simulink model "offboard_SSC_simscape"  (R2025b)
settings: Solver=ode23t  StartTime=0.0  StopTime=0.3  RelTol=1e-3
undefined symbols (not defined in the file): PLL_3ph__class, V_ref
libraries: fl_lib x39, nesl_utility x20, ee_lib x9, simulink x6, eeTransforms x2, batteryecm_lib x1, eeSinusoidalMeasurement x1
(part 1 of 2)
settings Model: SimulationMode=accelerator  Creator=a6039  LastModifiedBy=axz5845
settings SolverCC: AlgebraicLoopSolver=TrustRegion
settings DataIOCC: Decimation=50
settings DebuggingCC: SaveWithParameterizedLinksMsg=none  UnconnectedInputMsg=warning  UnconnectedOutputMsg=warning  UnconnectedLineMsg=warning
settings ModelReferenceCC: EnableRefExpFcnMdlSchedulingChecks=on
settings RTWCC: GPUComputeCapability=3.5  DLArmComputeVersion=19.05

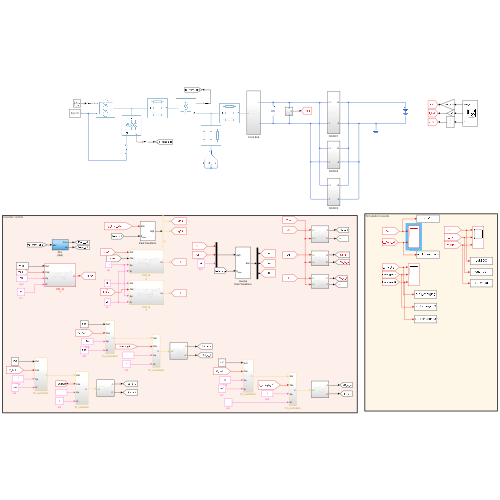
[thumbnail: Simulink's stored preview of the top-level diagram]
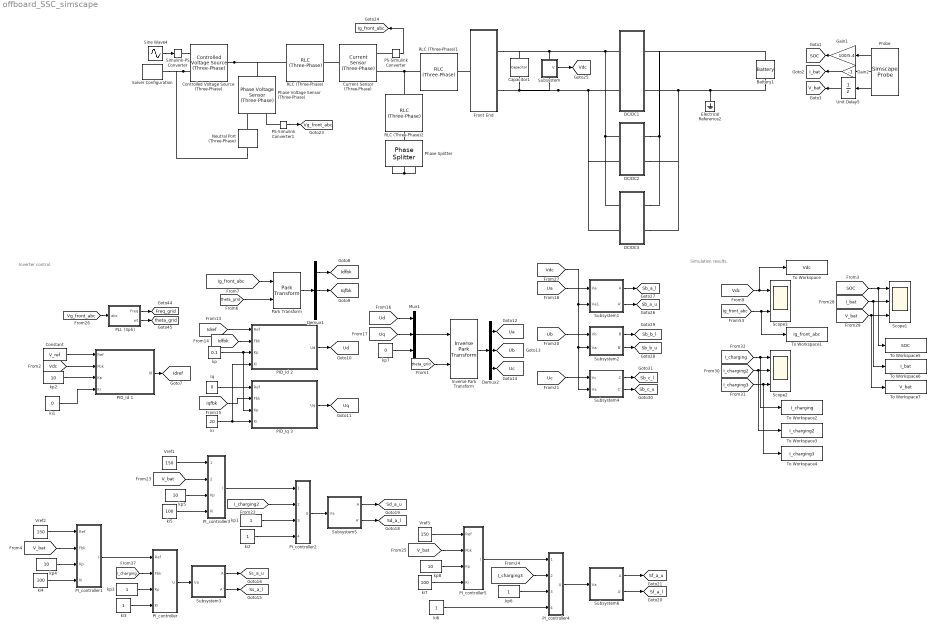
== system offboard_SSC_simscape ==
  note: Simulation results.
  note: Inverter control
  Battery1 : batteryecm_lib/Battery  Vnom=400 V  prm_dir=simscape.enum.battery.prm_dir.disabled  R1_dis=2 Ohm  R1_ch=2 Ohm  R1=2 Ohm  prm_AH=simscape.enum.battery.prm_AH.finite  AH=5.4 A*hr  V1=95 V  AH1=0.54 A*hr  prm_R2=simscape.enum.battery.prm_R2.disabled  R2=2000 Ohm  Tmeas=298.15 K  charge_measurement_port=simscape.enum.battery.enable.no  prm_dyn=simscape.enum.battery.prm_dyn.off  Rp1=0.005 Ohm  tau1=30 s  Rp2=0.005 Ohm  tau2=30 s  Rp3=0.005 Ohm  tau3=30 s  Rp4=0.005 Ohm  tau4=30 s  Rp5=0.005 Ohm  tau5=30 s  prm_fade=simscape.enum.battery.prm_fade.disabled  N_fade=100  AH_fade=45 A*hr  R1_fade=2.02 Ohm  R1_ch_fade=2.02 Ohm  V1_fade=10.35 V  prm_age=simscape.enum.battery.prm_age.disabled  prm_age_OCV=simscape.enum.battery.prm_age_OCV.OCV  OCV_age=0.9  SOC_age=60  Tmeas_age=298.15 K  delta_time_age_vec=[0] d  temperature_age_vec=[273] K  OCV_scaling_age=2.2134e6  OCV_offset_age=1.632e6  temp_exp_age=0.515833569 V  t_exp_age=0.75  Vnom_T2=12 V  R1_T2=2.2 Ohm  R1_T2_dis=2.2 Ohm  R1_T2_ch=2.2 Ohm  V1_T2=11.4 V  R2_T2=2200 Ohm  Rp1_T2=0.005 Ohm  tau1_T2=30 s  Rp2_T2=0.005 Ohm  tau2_T2=30 s  Rp3_T2=0.005 Ohm  tau3_T2=30 s  Rp4_T2=0.005 Ohm  tau4_T2=30 s  Rp5_T2=0.005 Ohm  tau5_T2=30 s  Tmeas2=273.15 K  thermal_port=simscape.enum.thermaleffects.omit  thermal_mass=30000 J/K  i_specify=off  i_priority=None  i=0 A  i_nominal_specify=off  i_nominal_value=1  i_nominal_unit=A  v_specify=off  v_priority=None  v=0 V  v_nominal_specify=off  v_nominal_value=1  v_nominal_unit=V  charge_specify=on  charge_priority=High  charge=0.54 A*hr  charge_nominal_specify=off  charge_nominal_value=1  charge_nominal_unit=A*hr  num_cycles_specify=off  num_cycles_priority=High  num_cycles=0  num_cycles_nominal_specify=off  num_cycles_nominal_value=1  num_cycles_nominal_unit=1  temperature_specify=off  temperature_priority=High  temperature=298.15 K  temperature_nominal_specify=off  temperature_nominal_value=1  temperature_nominal_unit=K
  Capacitor1 : fl_lib/Electrical/Electrical Elements/Capacitor  c=2 mF  r=1e-9 Ohm  g=0 1/Ohm  i_specify=off  i_priority=None  i=0 A  i_nominal_specify=off  i_nominal_value=1  i_nominal_unit=A  v_specify=off  v_priority=None  v=900 V  v_nominal_specify=off  v_nominal_value=1  v_nominal_unit=V  vc_specify=off  vc_priority=High  vc=900 V  vc_nominal_specify=off  vc_nominal_value=1  vc_nominal_unit=V
  Constant : Constant  Value=V_ref
  Controlled Voltage Source (Three-Phase) : ee_lib/Sources/Controlled Voltage Source (Three-Phase)  input_option=ee.enum.inputType.instantaneous  FRated=60 Hz
      settings: InternalSimscapePortConfiguration="{\"Bottom\":[],\"Left\":[{\"id\":\"S\",\"label\":\"S\",\"type\":\"input\"},{\"id\":\"n\",\"label\":\"n\",\"type\":\"foundation.electrical.electrical\"}],\"Right\":[{\"id\":\"N\",\"label\":\"~\",\"type\":\"foundation.electrical.three_phase\"}],\"Top\":[]}"
  Current Sensor (Three-Phase) : ee_lib/Sensors & Transducers/Current Sensor (Three-Phase)
  DC/DC1 : Subsystem
  DC/DC2 : Subsystem
  DC/DC3 : Subsystem
  Demux1 : Demux  Outputs=3
  Demux2 : Demux  Outputs=3
  Electrical Reference2 : fl_lib/Electrical/Electrical Elements/Electrical Reference
  Front End : Subsystem
  Gain1 : Gain  Gain=100/5.4
  Gain2 : Gain  Gain=-1
  Inverse Park Transform : eeTransforms/Inverse Park Transform  AxisAlignment=Q-axis  PowerInvariant=off
      settings: LibrarySourceBlock=|
      | ee_sl_lib/Mathematical
      | Transforms/Inverse
      | Park Transform
  Iq : Constant  Value=0
  Mux1 : Mux  Inputs=3
  Neutral Port (Three-Phase) : ee_lib/Connectors & References/Neutral Port (Three-Phase)  G_parasitic=1e-12 1/Ohm
      settings: InternalSimscapePortConfiguration="{\"Bottom\":[],\"Left\":[{\"id\":\"N\",\"label\":\"~\",\"type\":\"foundation.electrical.three_phase\"}],\"Right\":[{\"id\":\"n\",\"label\":\"n\",\"type\":\"foundation.electrical.electrical\"}],\"Top\":[]}"
  PID_Id 1 : Subsystem
  PID_Id 2 : Subsystem
  PID_Iq 3 : Subsystem
  PI_controller : Subsystem
  PI_controller1 : Subsystem
  PI_controller2 : Subsystem
  PI_controller3 : Subsystem
  PI_controller4 : Subsystem
  PI_controller5 : Subsystem
  PLL (3ph) : Subsystem
  PS-Simulink Converter : nesl_utility/PS-Simulink Converter  PhysicalDomain=network_engine_domain  SubClassName=ps_output  LeftPortType=input  RightPortType=output  PseudoPeriodic=off  Frequencies=[]  VectorFormat=inherit  Unit=inherit  AffineConversion=off
  PS-Simulink Converter1 : nesl_utility/PS-Simulink Converter  PhysicalDomain=network_engine_domain  SubClassName=ps_output  LeftPortType=input  RightPortType=output  PseudoPeriodic=off  Frequencies=[]  VectorFormat=inherit  Unit=inherit  AffineConversion=off
  Park Transform : eeTransforms/Park Transform  AxisAlignment=Q-axis  PowerInvariant=off
      settings: LibrarySourceBlock=|
      | ee_sl_lib/Mathematical
      | Transforms/Park Transform
  Phase Splitter : ee_lib/Connectors & References/Phase Splitter
  Phase Voltage Sensor (Three-Phase) : ee_lib/Sensors & Transducers/Phase Voltage Sensor (Three-Phase)
  Probe : SimscapeProbe  BoundBlock=1149  Variables="{\"charge\":{\"Probing\":\"ON\"},\"i\":{\"Probing\":\"ON\"},\"v\":{\"Probing\":\"ON\"}}"
  RLC (Three-Phase) : ee_lib/Passive/RLC Assemblies/RLC (Three-Phase)  port_option=ee.enum.threePhasePort.composite  component_structure=ee.enum.rlc.structure.SeriesRL  R=1 Ohm  L=1e-6 H  C=1e-6 F  R_parasitic=0 Ohm  G_parasitic=0 1/Ohm  IL_specify=off  IL_priority=High  IL=[0, 0, 0] A  IL_nominal_specify=off  IL_nominal_value=1  IL_nominal_unit=A  VC_specify=off  VC_priority=High  VC=[0, 0, 0] V  VC_nominal_specify=off  VC_nominal_value=1  VC_nominal_unit=V
      settings: InternalSimscapePortConfiguration="{\"Bottom\":[],\"Left\":[{\"id\":\"N1\",\"label\":\"~1\",\"type\":\"foundation.electrical.three_phase\"}],\"Right\":[{\"id\":\"N2\",\"label\":\"~2\",\"type\":\"foundation.electrical.three_phase\"}],\"Top\":[]}"
  RLC (Three-Phase)1 : ee_lib/Passive/RLC Assemblies/RLC (Three-Phase)  port_option=ee.enum.threePhasePort.composite  component_structure=ee.enum.rlc.structure.SeriesRL  R=1e-3 Ohm  L=250e-6 H  C=1e-6 F  R_parasitic=0 Ohm  G_parasitic=0 1/Ohm  IL_specify=off  IL_priority=High  IL=[0, 0, 0] A  IL_nominal_specify=off  IL_nominal_value=1  IL_nominal_unit=A  VC_specify=off  VC_priority=High  VC=[0, 0, 0] V  VC_nominal_specify=off  VC_nominal_value=1  VC_nominal_unit=V
      settings: InternalSimscapePortConfiguration="{\"Bottom\":[],\"Left\":[{\"id\":\"N1\",\"label\":\"~1\",\"type\":\"foundation.electrical.three_phase\"}],\"Right\":[{\"id\":\"N2\",\"label\":\"~2\",\"type\":\"foundation.electrical.three_phase\"}],\"Top\":[]}"
  RLC (Three-Phase)2 : ee_lib/Passive/RLC Assemblies/RLC (Three-Phase)  port_option=ee.enum.threePhasePort.composite  component_structure=ee.enum.rlc.structure.SeriesRC  R=1e-9 Ohm  L=80e-6 H  C=8.8e-6 F  R_parasitic=0 Ohm  G_parasitic=0 1/Ohm  IL_specify=off  IL_priority=High  IL=[0, 0, 0] A  IL_nominal_specify=off  IL_nominal_value=1  IL_nominal_unit=A  VC_specify=off  VC_priority=High  VC=[0, 0, 0] V  VC_nominal_specify=off  VC_nominal_value=1  VC_nominal_unit=V
      settings: InternalSimscapePortConfiguration="{\"Bottom\":[],\"Left\":[{\"id\":\"N1\",\"label\":\"~1\",\"type\":\"foundation.electrical.three_phase\"}],\"Right\":[{\"id\":\"N2\",\"label\":\"~2\",\"type\":\"foundation.electrical.three_phase\"}],\"Top\":[]}"
  Scope1 : Scope  NumInputPorts=3
      settings: ActiveDisplayYMinimum=9.9691692824175266  ActiveDisplayYMaximum=10.275296060537412
  Scope2 : Scope  NumInputPorts=3
      settings: ActiveDisplayYMinimum=-23.975369247286487  ActiveDisplayYMaximum=57.444989945022868  DataLoggingVariableName=ScopeData2
  Scope3 : Scope  NumInputPorts=2
      settings: ActiveDisplayYMinimum=885.40740395262992  ActiveDisplayYMaximum=897.78592526110128
  Simulink-PS Converter : nesl_utility/Simulink-PS Converter  PhysicalDomain=network_engine_domain  SubClassName=ps_input  LeftPortType=input  RightPortType=output  PseudoPeriodic=off  Frequencies=[]  NoiseDistribution=none  NoiseParameters=[]  Unit=1  AffineConversion=off  FilteringAndDerivatives=provide  SimscapeFilterOrder=1  InputFilterTimeConstant=0.001  UdotUserProvided=0
  Sine Wave4 : Sin  Amplitude=480  Frequency=60*2*pi  Phase=[0 -1 1]*2*pi/3  SampleTime=0
  Solver Configuration : nesl_utility/Solver Configuration  PhysicalDomain=network_engine_domain  SubClassName=solver  LeftPortType=input  RightPortType=generic  Tones=[]  Harmonics=[]  SimulateNoise=off  Profile=off  UseLocalSampling=off  EnableSwitchedLinearOptims=on  FrequencyDomain=off  UseCCode=off  RelTol=0.001  AbsTol=0.001  MinStep=1e-09  ToWorkspace=off  RevertToSquareIcSolve=off  NumHomotopyIterations=100  PhasorMode=off  PhasorModeNumHarmonics=1  ConsistencySolver=NEWTON_XTOL_AFTER_FTOL  IndexReductionMethod=DerivativeReplacement  DoDC=off  ResidualTolerance=1e-09  ConsistencyTolSource=GLOBAL  ConsistencyAbsTol=0.001  ConsistencyRelTol=0.001  ConsistencyTolFactor=0.001  UseLocalSolver=on  LocalSolverChoice=NE_BACKWARD_EULER_ADVANCER  ResolveIndetEquations=on  FunctionEvalNumThread=1  LocalSolverSampleTime=1e-6  DoFixedCost=on  MaxNonlinIter=2  MaxModeIter=2  ComputeImpulses=off  ImpulseIterations=2  LinearAlgebra=auto  LinearAlgebraNumThread=0  EquationFormulation=NE_TIME_EF  DelaysMemoryBudget=1024  AutomaticFiltering=off  FilteringTimeConstant=0.001  PartitionStorageMethod=AS_NEEDED  PartitionMemoryBudget=1024  PartitionMethod=ROBUST  MultibodyUseLocalSolver=off  MultibodyLocalSolverChoice=ODE1  MultibodyLocalSolverSampleTime=0.001
  Subsystem : Subsystem
      settings: PortSchema="{\"entries\":[{\"content\":{\"sides\":[{\"content\":{},\"type\":\"ConnectorPlacement.EquallySpacedRectSide\",\"uuid\":\"5292a83f-6f3d-4481-9274-991c3d86e7c3\"},{\"content\":{\"connectorIds\":[\"Out1\"],\"side\":\"RIGHT\"},\"type\":\"ConnectorPlacement.EquallySpacedRectSide\",\"uuid\":\"3f03e0e6-bee9-49df-bbfb-7f0a1aca1df7\"},{\"content\":{\"connectorIds\":[\"LConn1\"],\"side\":\"TOP\"},\"type\":\"ConnectorPlacement.EquallySpacedRectSide\",\"uuid\":\"842fbd6d-a974-4b26-821b-48593ae4fc83\"},{\"content\":{\"connectorIds\":[\"RConn1\"],\"side\":\"BOTTOM\"},\"type\":\"ConnectorPlacement.EquallySpacedRectSide\",\"uuid\":\"ab18bb4b-4bc5-4d22-a9fd-5b5abd0ee64f\"}]},\"type\":\"ConnectorPlacement.EquallySpacedConnector\",\"uuid\":\"a2f9b0d8-8bc3-4cf1-85b9-fb5408ef68da\"}],\"packageUris\":[\"http://schema.mathworks.com/mf0/Connector/R2020b\"],\"version\":\"1.0\"}"
  Subsystem1 : Subsystem
  Subsystem2 : Subsystem
  Subsystem3 : Subsystem
  Subsystem4 : Subsystem
  Subsystem5 : Subsystem
  Subsystem6 : Subsystem
  To Workspace : ToWorkspace  VariableName=Vdc  SaveFormat=Structure With Time  SampleTime=-1
  To Workspace1 : ToWorkspace  VariableName=Ig_front_abc  SaveFormat=Structure With Time  SampleTime=-1
  To Workspace2 : ToWorkspace  VariableName=I_charging  SaveFormat=Structure With Time  SampleTime=-1
  To Workspace3 : ToWorkspace  VariableName=I_charging2  SaveFormat=Structure With Time  SampleTime=-1
  To Workspace4 : ToWorkspace  VariableName=I_charging3  SaveFormat=Structure With Time  SampleTime=-1
  To Workspace5 : ToWorkspace  VariableName=SOC  SaveFormat=Structure With Time  SampleTime=-1
  To Workspace6 : ToWorkspace  VariableName=I_bat  SaveFormat=Structure With Time  SampleTime=-1
  To Workspace7 : ToWorkspace  VariableName=V_bat  SaveFormat=Structure With Time  SampleTime=-1
  Unit Delay5 : UnitDelay  SampleTime=-1  HasFrameUpgradeWarning=on
  Vref1 : Constant  Value=150
  Vref2 : Constant  Value=150
  Vref3 : Constant  Value=150
  ki : Constant  Value=20
  ki1 : Constant  Value=0
  ki2 : Constant
  ki3 : Constant
  ki4 : Constant  Value=100
  ki5 : Constant  Value=100
  ki6 : Constant
  ki7 : Constant  Value=100
  kp : Constant  Value=0.1
  kp1 : Constant
  kp{2,4..5,8} (4 alike) : Constant  Value=10
  kp3 : Constant
  kp6 : Constant
  kp7 : Constant  Value=0
  tag scope: Freq_grid=global, I_bat=global, Idfbk=global, Idref=global, Ig_front_abc=global, Iqfbk=global, SOC=global, Sb_a_l=global, Sb_a_u=global, Sb_b_l=global, Sb_b_u=global, Sb_c_l=global, Sb_c_u=global, Sd_a_l=global, Sd_a_u=global, Sf_a_l=global, Sf_a_u=global, Ss_a_l=global, Ss_a_u=global, Ua=global, Ub=global, Uc=global, Ud=global, Uq=global, V_bat=global, Vdc=global, Vg_front_abc=global, theta_grid=global
  wires:
  Demux2/3 -> [Uc]
  ki1/1 -> PID_Id 1/4(Ki)
  Demux2/1 -> [Ua]
  [theta_grid] -> Inverse Park Transform/2
  Demux2/2 -> [Ub]
  [Uq] -> Mux1/2
  [Ua] -> Subsystem1/1(Va)
  [Idfbk] -> PID_Id 2/2(Fbk)
  Demux1/1 -> [Idfbk]
  PID_Id 1/1(Id) -> [Idref]
  kp7/1 -> Mux1/3
  PID_Id 2/1(Ud) -> [Ud]
  PID_Iq 3/1(Uq) -> [Uq]
  [Ud] -> Mux1/1
  [Uc] -> Subsystem4/1(Vc)
  [Iqfbk] -> PID_Iq 3/2(Fbk)
  ki/1 -> PID_Id 2/4(Ki), PID_Iq 3/4(Ki)
  [Ig_front_abc] -> Park Transform/1
  [Ub] -> Subsystem2/1(Vb)
  Inverse Park Transform/1 -> Demux2/1
  Park Transform/1 -> Demux1/1
  kp/1 -> PID_Iq 3/3(Kp), PID_Id 2/3(Kp)
  [theta_grid] -> Park Transform/2
  kp2/1 -> PID_Id 1/3(Kp)
  Subsystem1/2(A') -> [Sb_a_u]
  Subsystem1/1(A) -> [Sb_a_l]
  Subsystem2/2(B') -> [Sb_b_u]
  Subsystem2/1(B) -> [Sb_b_l]
  Subsystem4/2(C') -> [Sb_c_u]
  Subsystem4/1(C) -> [Sb_c_l]
  [Ig_front_abc] -> To Workspace1/1, Scope3/2
  [Vdc] -> To Workspace/1, Scope3/1
  [I_charging] -> PI_controller/2(Fbk)
  [V_bat] -> PI_controller1/2(Fbk)
  kp4/1 -> PI_controller1/3(Kp)
  ki3/1 -> PI_controller/4(Ki)
  ki4/1 -> PI_controller1/4(Ki)
  Vref2/1 -> PI_controller1/1(Ref)
  kp3/1 -> PI_controller/3(Kp)
  PI_controller/1(U) -> Subsystem3/1(Va)
  Subsystem3/1(A) -> [Ss_a_u]
  Subsystem3/2(A') -> [Ss_a_l]
  Subsystem5/1(A) -> [Sd_a_u]
  Subsystem5/2(A') -> [Sd_a_l]
  PI_controller2/1(U) -> Subsystem5/1(Va)
  ki5/1 -> PI_controller3/4(Ki)
  ki2/1 -> PI_controller2/4(Ki)
  Vref1/1 -> PI_controller3/1(Ref)
  kp1/1 -> PI_controller2/3(Kp)
  kp5/1 -> PI_controller3/3(Kp)
  [I_charging2] -> PI_controller2/2(Fbk)
  [V_bat] -> PI_controller3/2(Fbk)
  Subsystem6/1(A) -> [Sf_a_u]
  Subsystem6/2(A') -> [Sf_a_l]
  PI_controller4/1(U) -> Subsystem6/1(Va)
  ki7/1 -> PI_controller5/4(Ki)
  ki6/1 -> PI_controller4/4(Ki)
  Vref3/1 -> PI_controller5/1(Ref)
  kp6/1 -> PI_controller4/3(Kp)
  kp8/1 -> PI_controller5/3(Kp)
  [I_charging3] -> PI_controller4/2(Fbk)
  [V_bat] -> PI_controller5/2(Fbk)
  PI_controller1/1(I) -> PI_controller/1(Ref)
  PI_controller3/1(I) -> PI_controller2/1(Ref)
  PI_controller5/1(I) -> PI_controller4/1(Ref)
  [Vg_front_abc] -> PLL (3ph)/1(abc)
  PLL (3ph)/1(Freq) -> [Freq_grid]
  PLL (3ph)/2(wt) -> [theta_grid]
  [Vdc] -> Subsystem4/2(Va), Subsystem2/2(Va), Subsystem1/2(Va1)
  [SOC] -> To Workspace5/1, Scope1/1
  [I_bat] -> To Workspace6/1, Scope1/2
  [V_bat] -> To Workspace7/1, Scope1/3
  [I_charging] -> To Workspace2/1, Scope2/1
  [I_charging2] -> To Workspace3/1, Scope2/2
  [I_charging3] -> To Workspace4/1, Scope2/3
  PS-Simulink Converter1/1 -> [Vg_front_abc]
  PS-Simulink Converter/1 -> [Ig_front_abc]
  Subsystem/1(V) -> [Vdc]
  Sine Wave4/1 -> Simulink-PS Converter/1
  Mux1/1 -> Inverse Park Transform/1
  Probe/3 -> Unit Delay5/1
  Probe/2 -> Gain2/1
  Probe/1 -> Gain1/1
  Gain1/1 -> [SOC]
  Unit Delay5/1 -> [V_bat]
  Gain2/1 -> [I_bat]
  [Vdc] -> PID_Id 1/2(Fbk)
  Constant/1 -> PID_Id 1/1(Ref)
  [Idref] -> PID_Id 2/1(Ref)
  Iq/1 -> PID_Iq 3/1(Ref)
  Demux1/2 -> [Iqfbk]
  connections:
  RLC (Three-Phase)2/LConn1 -- RLC (Three-Phase)1/LConn1 -- Current Sensor (Three-Phase)/RConn2
  Controlled Voltage Source (Three-Phase)/RConn1 -- RLC (Three-Phase)/LConn1 -- Phase Voltage Sensor (Three-Phase)/LConn1
  Controlled Voltage Source (Three-Phase)/LConn2 -- Neutral Port (Three-Phase)/RConn1 -- Solver Configuration/RConn1
  Neutral Port (Three-Phase)/LConn1 -- Phase Voltage Sensor (Three-Phase)/RConn2
  Front End/LConn1 -- RLC (Three-Phase)1/RConn1
  PS-Simulink Converter1/LConn1 -- Phase Voltage Sensor (Three-Phase)/RConn1
  Phase Splitter/LConn1 -- RLC (Three-Phase)2/RConn1
  PS-Simulink Converter/LConn1 -- Current Sensor (Three-Phase)/RConn1
  Current Sensor (Three-Phase)/LConn1 -- RLC (Three-Phase)/RConn1
  Simulink-PS Converter/RConn1 -- Controlled Voltage Source (Three-Phase)/LConn1
  Phase Splitter/RConn1 -- Phase Splitter/RConn2 -- Phase Splitter/RConn3
  Capacitor1/RConn1 -- Subsystem/RConn1 -- DC/DC1/LConn2 -- DC/DC3/LConn2 -- DC/DC2/LConn2 -- Front End/RConn2
  DC/DC2/RConn1 -- DC/DC3/RConn1 -- DC/DC1/RConn1 -- Battery1/LConn1
  DC/DC2/LConn1 -- DC/DC3/LConn1 -- Subsystem/LConn1 -- Capacitor1/LConn1 -- Front End/RConn1 -- DC/DC1/LConn1
  Battery1/RConn1 -- Electrical Reference2/LConn1 -- DC/DC3/RConn2 -- DC/DC2/RConn2 -- DC/DC1/RConn2

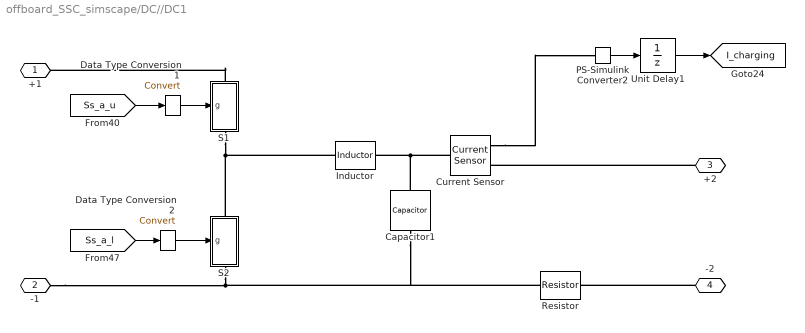
== system offboard_SSC_simscape/DC//DC1 ==
  Capacitor1 : fl_lib/Electrical/Electrical Elements/Capacitor  c=500e-6 F  r=1e-9 Ohm  g=0 1/Ohm  i_specify=off  i_priority=None  i=0 A  i_nominal_specify=off  i_nominal_value=1  i_nominal_unit=A  v_specify=off  v_priority=None  v=0 V  v_nominal_specify=off  v_nominal_value=1  v_nominal_unit=V  vc_specify=off  vc_priority=High  vc=0 V  vc_nominal_specify=off  vc_nominal_value=1  vc_nominal_unit=V
  Current Sensor : fl_lib/Electrical/Electrical Sensors/Current Sensor
  Data Type Conversion1 : DataTypeConversion  SaturateOnIntegerOverflow=off  RndMeth=Floor
  Data Type Conversion2 : DataTypeConversion  SaturateOnIntegerOverflow=off  RndMeth=Floor
  Inductor : fl_lib/Electrical/Electrical Elements/Inductor  l=10e-6 H  r=0 Ohm  g=0 1/Ohm  i_specify=off  i_priority=None  i=0 A  i_nominal_specify=off  i_nominal_value=1  i_nominal_unit=A  v_specify=off  v_priority=None  v=0 V  v_nominal_specify=off  v_nominal_value=1  v_nominal_unit=V  i_L_specify=off  i_L_priority=High  i_L=0 A  i_L_nominal_specify=off  i_L_nominal_value=1  i_L_nominal_unit=A
  PS-Simulink Converter2 : nesl_utility/PS-Simulink Converter  PhysicalDomain=network_engine_domain  SubClassName=ps_output  LeftPortType=input  RightPortType=output  PseudoPeriodic=off  Frequencies=[]  VectorFormat=inherit  Unit=inherit  AffineConversion=off
  Resistor : fl_lib/Electrical/Electrical Elements/Resistor  R=1e-9 Ohm  i_specify=off  i_priority=None  i=0 A  i_nominal_specify=off  i_nominal_value=1  i_nominal_unit=A  v_specify=off  v_priority=None  v=0 V  v_nominal_specify=off  v_nominal_value=1  v_nominal_unit=V
  S1 : Subsystem
      settings: PortSchema="{\"entries\":[{\"content\":{\"sides\":[{\"content\":{\"connectorIds\":[\"In1\"]},\"type\":\"ConnectorPlacement.EquallySpacedRectSide\",\"uuid\":\"4868c43b-8f86-4e2f-a4da-367c2e17d6e4\"},{\"content\":{\"side\":\"RIGHT\"},\"type\":\"ConnectorPlacement.EquallySpacedRectSide\",\"uuid\":\"ebe9b5ec-833b-4a08-98e5-ff684cd7afcb\"},{\"content\":{\"connectorIds\":[\"LConn1\"],\"side\":\"TOP\"},\"type\":\"ConnectorPlacement.EquallySpacedRectSide\",\"uuid\":\"c72df866-8baa-41a8-9bb1-42a4a1fdee71\"},{\"content\":{\"connectorIds\":[\"RConn1\"],\"side\":\"BOTTOM\"},\"type\":\"ConnectorPlacement.EquallySpacedRectSide\",\"uuid\":\"3a9867c5-1563-48cb-a4f4-92deec85fd3d\"}]},\"type\":\"ConnectorPlacement.EquallySpacedConnector\",\"uuid\":\"206e0d7b-1d35-45e7-9c4c-8a6f9fe9dc79\"}],\"packageUris\":[\"http://schema.mathworks.com/mf0/Connector/R2020b\"],\"version\":\"1.0\"}"
  S2 : Subsystem
      settings: PortSchema="{\"entries\":[{\"content\":{\"sides\":[{\"content\":{\"connectorIds\":[\"In1\"]},\"type\":\"ConnectorPlacement.EquallySpacedRectSide\",\"uuid\":\"4868c43b-8f86-4e2f-a4da-367c2e17d6e4\"},{\"content\":{\"side\":\"RIGHT\"},\"type\":\"ConnectorPlacement.EquallySpacedRectSide\",\"uuid\":\"ebe9b5ec-833b-4a08-98e5-ff684cd7afcb\"},{\"content\":{\"connectorIds\":[\"LConn1\"],\"side\":\"TOP\"},\"type\":\"ConnectorPlacement.EquallySpacedRectSide\",\"uuid\":\"c72df866-8baa-41a8-9bb1-42a4a1fdee71\"},{\"content\":{\"connectorIds\":[\"RConn1\"],\"side\":\"BOTTOM\"},\"type\":\"ConnectorPlacement.EquallySpacedRectSide\",\"uuid\":\"3a9867c5-1563-48cb-a4f4-92deec85fd3d\"}]},\"type\":\"ConnectorPlacement.EquallySpacedConnector\",\"uuid\":\"206e0d7b-1d35-45e7-9c4c-8a6f9fe9dc79\"}],\"packageUris\":[\"http://schema.mathworks.com/mf0/Connector/R2020b\"],\"version\":\"1.0\"}"
  Unit Delay1 : UnitDelay  SampleTime=-1  HasFrameUpgradeWarning=on
  +1 : PMIOPort  Side=Left
  -1 : PMIOPort  Port=2  Side=Left
  +2 : PMIOPort  Port=3  Side=Right
  -2 : PMIOPort  Port=4  Side=Right
  tag scope: I_charging=global
  wires:
  [Ss_a_l] -> Data Type Conversion2/1
  PS-Simulink Converter2/1 -> Unit Delay1/1
  [Ss_a_u] -> Data Type Conversion1/1
  Data Type Conversion1/1 -> S1/1(g)
  Data Type Conversion2/1 -> S2/1(g)
  Unit Delay1/1 -> [I_charging]
  connections:
  Inductor/LConn1 -- S2/LConn1 -- S1/RConn1
  S1/LConn1 -- +1/RConn1
  Current Sensor/RConn1 -- PS-Simulink Converter2/LConn1
  -1/RConn1 -- S2/RConn1 -- Resistor/LConn1 -- Capacitor1/RConn1
  Capacitor1/LConn1 -- Inductor/RConn1 -- Current Sensor/LConn1
  +2/RConn1 -- Current Sensor/RConn2
  -2/RConn1 -- Resistor/RConn1

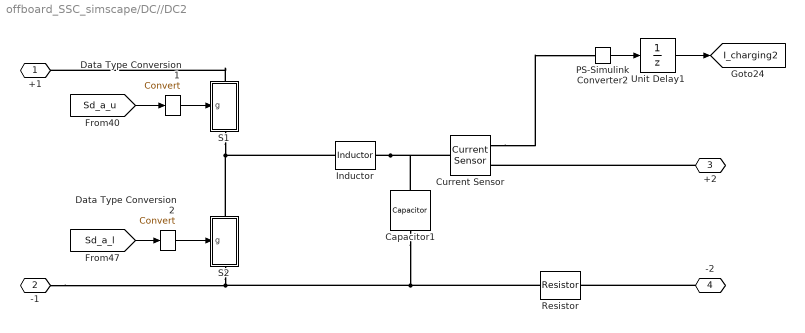
== system offboard_SSC_simscape/DC//DC2 ==
  Capacitor1 : fl_lib/Electrical/Electrical Elements/Capacitor  c=500e-6 F  r=1e-9 Ohm  g=0 1/Ohm  i_specify=off  i_priority=None  i=0 A  i_nominal_specify=off  i_nominal_value=1  i_nominal_unit=A  v_specify=off  v_priority=None  v=0 V  v_nominal_specify=off  v_nominal_value=1  v_nominal_unit=V  vc_specify=off  vc_priority=High  vc=0 V  vc_nominal_specify=off  vc_nominal_value=1  vc_nominal_unit=V
  Current Sensor : fl_lib/Electrical/Electrical Sensors/Current Sensor
  Data Type Conversion1 : DataTypeConversion  SaturateOnIntegerOverflow=off  RndMeth=Floor
  Data Type Conversion2 : DataTypeConversion  SaturateOnIntegerOverflow=off  RndMeth=Floor
  Inductor : fl_lib/Electrical/Electrical Elements/Inductor  l=10e-6 H  r=0 Ohm  g=0 1/Ohm  i_specify=off  i_priority=None  i=0 A  i_nominal_specify=off  i_nominal_value=1  i_nominal_unit=A  v_specify=off  v_priority=None  v=0 V  v_nominal_specify=off  v_nominal_value=1  v_nominal_unit=V  i_L_specify=off  i_L_priority=High  i_L=0 A  i_L_nominal_specify=off  i_L_nominal_value=1  i_L_nominal_unit=A
  PS-Simulink Converter2 : nesl_utility/PS-Simulink Converter  PhysicalDomain=network_engine_domain  SubClassName=ps_output  LeftPortType=input  RightPortType=output  PseudoPeriodic=off  Frequencies=[]  VectorFormat=inherit  Unit=inherit  AffineConversion=off
  Resistor : fl_lib/Electrical/Electrical Elements/Resistor  R=1e-9 Ohm  i_specify=off  i_priority=None  i=0 A  i_nominal_specify=off  i_nominal_value=1  i_nominal_unit=A  v_specify=off  v_priority=None  v=0 V  v_nominal_specify=off  v_nominal_value=1  v_nominal_unit=V
  S1 : Subsystem
      settings: PortSchema="{\"entries\":[{\"content\":{\"sides\":[{\"content\":{\"connectorIds\":[\"In1\"]},\"type\":\"ConnectorPlacement.EquallySpacedRectSide\",\"uuid\":\"4868c43b-8f86-4e2f-a4da-367c2e17d6e4\"},{\"content\":{\"side\":\"RIGHT\"},\"type\":\"ConnectorPlacement.EquallySpacedRectSide\",\"uuid\":\"ebe9b5ec-833b-4a08-98e5-ff684cd7afcb\"},{\"content\":{\"connectorIds\":[\"LConn1\"],\"side\":\"TOP\"},\"type\":\"ConnectorPlacement.EquallySpacedRectSide\",\"uuid\":\"c72df866-8baa-41a8-9bb1-42a4a1fdee71\"},{\"content\":{\"connectorIds\":[\"RConn1\"],\"side\":\"BOTTOM\"},\"type\":\"ConnectorPlacement.EquallySpacedRectSide\",\"uuid\":\"3a9867c5-1563-48cb-a4f4-92deec85fd3d\"}]},\"type\":\"ConnectorPlacement.EquallySpacedConnector\",\"uuid\":\"206e0d7b-1d35-45e7-9c4c-8a6f9fe9dc79\"}],\"packageUris\":[\"http://schema.mathworks.com/mf0/Connector/R2020b\"],\"version\":\"1.0\"}"
  S2 : Subsystem
      settings: PortSchema="{\"entries\":[{\"content\":{\"sides\":[{\"content\":{\"connectorIds\":[\"In1\"]},\"type\":\"ConnectorPlacement.EquallySpacedRectSide\",\"uuid\":\"4868c43b-8f86-4e2f-a4da-367c2e17d6e4\"},{\"content\":{\"side\":\"RIGHT\"},\"type\":\"ConnectorPlacement.EquallySpacedRectSide\",\"uuid\":\"ebe9b5ec-833b-4a08-98e5-ff684cd7afcb\"},{\"content\":{\"connectorIds\":[\"LConn1\"],\"side\":\"TOP\"},\"type\":\"ConnectorPlacement.EquallySpacedRectSide\",\"uuid\":\"c72df866-8baa-41a8-9bb1-42a4a1fdee71\"},{\"content\":{\"connectorIds\":[\"RConn1\"],\"side\":\"BOTTOM\"},\"type\":\"ConnectorPlacement.EquallySpacedRectSide\",\"uuid\":\"3a9867c5-1563-48cb-a4f4-92deec85fd3d\"}]},\"type\":\"ConnectorPlacement.EquallySpacedConnector\",\"uuid\":\"206e0d7b-1d35-45e7-9c4c-8a6f9fe9dc79\"}],\"packageUris\":[\"http://schema.mathworks.com/mf0/Connector/R2020b\"],\"version\":\"1.0\"}"
  Unit Delay1 : UnitDelay  SampleTime=-1  HasFrameUpgradeWarning=on
  +1 : PMIOPort  Side=Left
  -1 : PMIOPort  Port=2  Side=Left
  +2 : PMIOPort  Port=3  Side=Right
  -2 : PMIOPort  Port=4  Side=Right
  tag scope: I_charging2=global
  wires:
  Unit Delay1/1 -> [I_charging2]
  Data Type Conversion2/1 -> S2/1(g)
  Data Type Conversion1/1 -> S1/1(g)
  [Sd_a_u] -> Data Type Conversion1/1
  PS-Simulink Converter2/1 -> Unit Delay1/1
  [Sd_a_l] -> Data Type Conversion2/1
  connections:
  -2/RConn1 -- Resistor/RConn1
  +2/RConn1 -- Current Sensor/RConn2
  Inductor/RConn1 -- Capacitor1/LConn1 -- Current Sensor/LConn1
  Resistor/LConn1 -- Capacitor1/RConn1 -- S2/RConn1 -- -1/RConn1
  Current Sensor/RConn1 -- PS-Simulink Converter2/LConn1
  S1/LConn1 -- +1/RConn1
  Inductor/LConn1 -- S2/LConn1 -- S1/RConn1

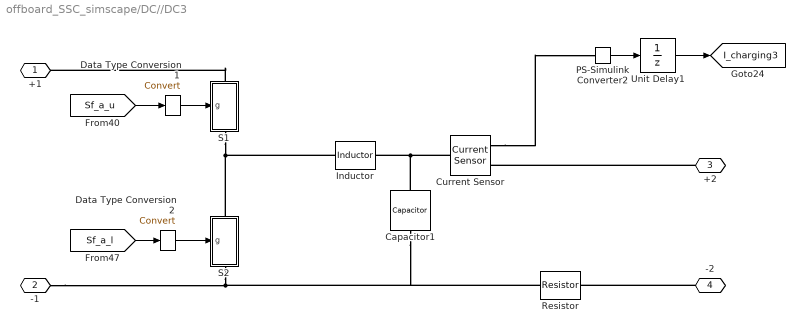
== system offboard_SSC_simscape/DC//DC3 ==
  Capacitor1 : fl_lib/Electrical/Electrical Elements/Capacitor  c=500e-6 F  r=1e-9 Ohm  g=0 1/Ohm  i_specify=off  i_priority=None  i=0 A  i_nominal_specify=off  i_nominal_value=1  i_nominal_unit=A  v_specify=off  v_priority=None  v=0 V  v_nominal_specify=off  v_nominal_value=1  v_nominal_unit=V  vc_specify=off  vc_priority=High  vc=0 V  vc_nominal_specify=off  vc_nominal_value=1  vc_nominal_unit=V
  Current Sensor : fl_lib/Electrical/Electrical Sensors/Current Sensor
  Data Type Conversion1 : DataTypeConversion  SaturateOnIntegerOverflow=off  RndMeth=Floor
  Data Type Conversion2 : DataTypeConversion  SaturateOnIntegerOverflow=off  RndMeth=Floor
  Inductor : fl_lib/Electrical/Electrical Elements/Inductor  l=10e-6 H  r=0 Ohm  g=0 1/Ohm  i_specify=off  i_priority=None  i=0 A  i_nominal_specify=off  i_nominal_value=1  i_nominal_unit=A  v_specify=off  v_priority=None  v=0 V  v_nominal_specify=off  v_nominal_value=1  v_nominal_unit=V  i_L_specify=off  i_L_priority=High  i_L=0 A  i_L_nominal_specify=off  i_L_nominal_value=1  i_L_nominal_unit=A
  PS-Simulink Converter2 : nesl_utility/PS-Simulink Converter  PhysicalDomain=network_engine_domain  SubClassName=ps_output  LeftPortType=input  RightPortType=output  PseudoPeriodic=off  Frequencies=[]  VectorFormat=inherit  Unit=inherit  AffineConversion=off
  Resistor : fl_lib/Electrical/Electrical Elements/Resistor  R=1e-9 Ohm  i_specify=off  i_priority=None  i=0 A  i_nominal_specify=off  i_nominal_value=1  i_nominal_unit=A  v_specify=off  v_priority=None  v=0 V  v_nominal_specify=off  v_nominal_value=1  v_nominal_unit=V
  S1 : Subsystem
      settings: PortSchema="{\"entries\":[{\"content\":{\"sides\":[{\"content\":{\"connectorIds\":[\"In1\"]},\"type\":\"ConnectorPlacement.EquallySpacedRectSide\",\"uuid\":\"4868c43b-8f86-4e2f-a4da-367c2e17d6e4\"},{\"content\":{\"side\":\"RIGHT\"},\"type\":\"ConnectorPlacement.EquallySpacedRectSide\",\"uuid\":\"ebe9b5ec-833b-4a08-98e5-ff684cd7afcb\"},{\"content\":{\"connectorIds\":[\"LConn1\"],\"side\":\"TOP\"},\"type\":\"ConnectorPlacement.EquallySpacedRectSide\",\"uuid\":\"c72df866-8baa-41a8-9bb1-42a4a1fdee71\"},{\"content\":{\"connectorIds\":[\"RConn1\"],\"side\":\"BOTTOM\"},\"type\":\"ConnectorPlacement.EquallySpacedRectSide\",\"uuid\":\"3a9867c5-1563-48cb-a4f4-92deec85fd3d\"}]},\"type\":\"ConnectorPlacement.EquallySpacedConnector\",\"uuid\":\"206e0d7b-1d35-45e7-9c4c-8a6f9fe9dc79\"}],\"packageUris\":[\"http://schema.mathworks.com/mf0/Connector/R2020b\"],\"version\":\"1.0\"}"
  S2 : Subsystem
      settings: PortSchema="{\"entries\":[{\"content\":{\"sides\":[{\"content\":{\"connectorIds\":[\"In1\"]},\"type\":\"ConnectorPlacement.EquallySpacedRectSide\",\"uuid\":\"4868c43b-8f86-4e2f-a4da-367c2e17d6e4\"},{\"content\":{\"side\":\"RIGHT\"},\"type\":\"ConnectorPlacement.EquallySpacedRectSide\",\"uuid\":\"ebe9b5ec-833b-4a08-98e5-ff684cd7afcb\"},{\"content\":{\"connectorIds\":[\"LConn1\"],\"side\":\"TOP\"},\"type\":\"ConnectorPlacement.EquallySpacedRectSide\",\"uuid\":\"c72df866-8baa-41a8-9bb1-42a4a1fdee71\"},{\"content\":{\"connectorIds\":[\"RConn1\"],\"side\":\"BOTTOM\"},\"type\":\"ConnectorPlacement.EquallySpacedRectSide\",\"uuid\":\"3a9867c5-1563-48cb-a4f4-92deec85fd3d\"}]},\"type\":\"ConnectorPlacement.EquallySpacedConnector\",\"uuid\":\"206e0d7b-1d35-45e7-9c4c-8a6f9fe9dc79\"}],\"packageUris\":[\"http://schema.mathworks.com/mf0/Connector/R2020b\"],\"version\":\"1.0\"}"
  Unit Delay1 : UnitDelay  SampleTime=-1  HasFrameUpgradeWarning=on
  +1 : PMIOPort  Side=Left
  -1 : PMIOPort  Port=2  Side=Left
  +2 : PMIOPort  Port=3  Side=Right
  -2 : PMIOPort  Port=4  Side=Right
  tag scope: I_charging3=global
  wires:
  [Sf_a_l] -> Data Type Conversion2/1
  PS-Simulink Converter2/1 -> Unit Delay1/1
  [Sf_a_u] -> Data Type Conversion1/1
  Data Type Conversion1/1 -> S1/1(g)
  Data Type Conversion2/1 -> S2/1(g)
  Unit Delay1/1 -> [I_charging3]
  connections:
  Inductor/LConn1 -- S2/LConn1 -- S1/RConn1
  S1/LConn1 -- +1/RConn1
  Current Sensor/RConn1 -- PS-Simulink Converter2/LConn1
  -1/RConn1 -- S2/RConn1 -- Capacitor1/RConn1 -- Resistor/LConn1
  Current Sensor/LConn1 -- Capacitor1/LConn1 -- Inductor/RConn1
  +2/RConn1 -- Current Sensor/RConn2
  -2/RConn1 -- Resistor/RConn1

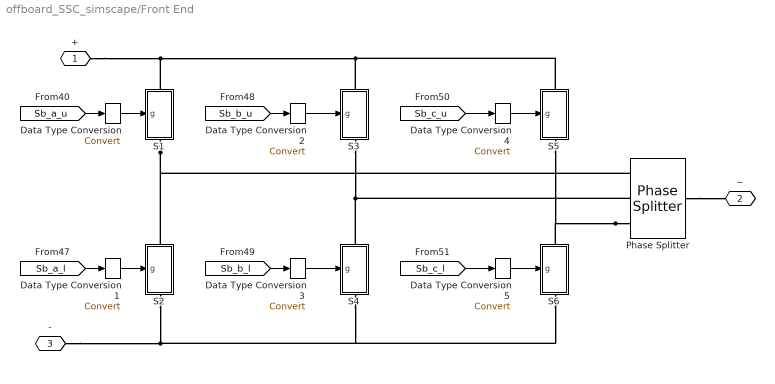
== system offboard_SSC_simscape/Front End ==
  Data Type Conversion{,1..5} (6 alike) : DataTypeConversion  SaturateOnIntegerOverflow=off  RndMeth=Floor
  Phase Splitter : ee_lib/Connectors & References/Phase Splitter
  S1 : Subsystem
      settings: PortSchema="{\"entries\":[{\"content\":{\"sides\":[{\"content\":{\"connectorIds\":[\"In1\"]},\"type\":\"ConnectorPlacement.EquallySpacedRectSide\",\"uuid\":\"4868c43b-8f86-4e2f-a4da-367c2e17d6e4\"},{\"content\":{\"side\":\"RIGHT\"},\"type\":\"ConnectorPlacement.EquallySpacedRectSide\",\"uuid\":\"ebe9b5ec-833b-4a08-98e5-ff684cd7afcb\"},{\"content\":{\"connectorIds\":[\"LConn1\"],\"side\":\"TOP\"},\"type\":\"ConnectorPlacement.EquallySpacedRectSide\",\"uuid\":\"c72df866-8baa-41a8-9bb1-42a4a1fdee71\"},{\"content\":{\"connectorIds\":[\"RConn1\"],\"side\":\"BOTTOM\"},\"type\":\"ConnectorPlacement.EquallySpacedRectSide\",\"uuid\":\"3a9867c5-1563-48cb-a4f4-92deec85fd3d\"}]},\"type\":\"ConnectorPlacement.EquallySpacedConnector\",\"uuid\":\"206e0d7b-1d35-45e7-9c4c-8a6f9fe9dc79\"}],\"packageUris\":[\"http://schema.mathworks.com/mf0/Connector/R2020b\"],\"version\":\"1.0\"}"
  S2 : Subsystem
      settings: PortSchema="{\"entries\":[{\"content\":{\"sides\":[{\"content\":{\"connectorIds\":[\"In1\"]},\"type\":\"ConnectorPlacement.EquallySpacedRectSide\",\"uuid\":\"4868c43b-8f86-4e2f-a4da-367c2e17d6e4\"},{\"content\":{\"side\":\"RIGHT\"},\"type\":\"ConnectorPlacement.EquallySpacedRectSide\",\"uuid\":\"ebe9b5ec-833b-4a08-98e5-ff684cd7afcb\"},{\"content\":{\"connectorIds\":[\"LConn1\"],\"side\":\"TOP\"},\"type\":\"ConnectorPlacement.EquallySpacedRectSide\",\"uuid\":\"c72df866-8baa-41a8-9bb1-42a4a1fdee71\"},{\"content\":{\"connectorIds\":[\"RConn1\"],\"side\":\"BOTTOM\"},\"type\":\"ConnectorPlacement.EquallySpacedRectSide\",\"uuid\":\"3a9867c5-1563-48cb-a4f4-92deec85fd3d\"}]},\"type\":\"ConnectorPlacement.EquallySpacedConnector\",\"uuid\":\"206e0d7b-1d35-45e7-9c4c-8a6f9fe9dc79\"}],\"packageUris\":[\"http://schema.mathworks.com/mf0/Connector/R2020b\"],\"version\":\"1.0\"}"
  S3 : Subsystem
      settings: PortSchema="{\"entries\":[{\"content\":{\"sides\":[{\"content\":{\"connectorIds\":[\"In1\"]},\"type\":\"ConnectorPlacement.EquallySpacedRectSide\",\"uuid\":\"4868c43b-8f86-4e2f-a4da-367c2e17d6e4\"},{\"content\":{\"side\":\"RIGHT\"},\"type\":\"ConnectorPlacement.EquallySpacedRectSide\",\"uuid\":\"ebe9b5ec-833b-4a08-98e5-ff684cd7afcb\"},{\"content\":{\"connectorIds\":[\"LConn1\"],\"side\":\"TOP\"},\"type\":\"ConnectorPlacement.EquallySpacedRectSide\",\"uuid\":\"c72df866-8baa-41a8-9bb1-42a4a1fdee71\"},{\"content\":{\"connectorIds\":[\"RConn1\"],\"side\":\"BOTTOM\"},\"type\":\"ConnectorPlacement.EquallySpacedRectSide\",\"uuid\":\"3a9867c5-1563-48cb-a4f4-92deec85fd3d\"}]},\"type\":\"ConnectorPlacement.EquallySpacedConnector\",\"uuid\":\"206e0d7b-1d35-45e7-9c4c-8a6f9fe9dc79\"}],\"packageUris\":[\"http://schema.mathworks.com/mf0/Connector/R2020b\"],\"version\":\"1.0\"}"
  S4 : Subsystem
      settings: PortSchema="{\"entries\":[{\"content\":{\"sides\":[{\"content\":{\"connectorIds\":[\"In1\"]},\"type\":\"ConnectorPlacement.EquallySpacedRectSide\",\"uuid\":\"4868c43b-8f86-4e2f-a4da-367c2e17d6e4\"},{\"content\":{\"side\":\"RIGHT\"},\"type\":\"ConnectorPlacement.EquallySpacedRectSide\",\"uuid\":\"ebe9b5ec-833b-4a08-98e5-ff684cd7afcb\"},{\"content\":{\"connectorIds\":[\"LConn1\"],\"side\":\"TOP\"},\"type\":\"ConnectorPlacement.EquallySpacedRectSide\",\"uuid\":\"c72df866-8baa-41a8-9bb1-42a4a1fdee71\"},{\"content\":{\"connectorIds\":[\"RConn1\"],\"side\":\"BOTTOM\"},\"type\":\"ConnectorPlacement.EquallySpacedRectSide\",\"uuid\":\"3a9867c5-1563-48cb-a4f4-92deec85fd3d\"}]},\"type\":\"ConnectorPlacement.EquallySpacedConnector\",\"uuid\":\"206e0d7b-1d35-45e7-9c4c-8a6f9fe9dc79\"}],\"packageUris\":[\"http://schema.mathworks.com/mf0/Connector/R2020b\"],\"version\":\"1.0\"}"
  S5 : Subsystem
      settings: PortSchema="{\"entries\":[{\"content\":{\"sides\":[{\"content\":{\"connectorIds\":[\"In1\"]},\"type\":\"ConnectorPlacement.EquallySpacedRectSide\",\"uuid\":\"4868c43b-8f86-4e2f-a4da-367c2e17d6e4\"},{\"content\":{\"side\":\"RIGHT\"},\"type\":\"ConnectorPlacement.EquallySpacedRectSide\",\"uuid\":\"ebe9b5ec-833b-4a08-98e5-ff684cd7afcb\"},{\"content\":{\"connectorIds\":[\"LConn1\"],\"side\":\"TOP\"},\"type\":\"ConnectorPlacement.EquallySpacedRectSide\",\"uuid\":\"c72df866-8baa-41a8-9bb1-42a4a1fdee71\"},{\"content\":{\"connectorIds\":[\"RConn1\"],\"side\":\"BOTTOM\"},\"type\":\"ConnectorPlacement.EquallySpacedRectSide\",\"uuid\":\"3a9867c5-1563-48cb-a4f4-92deec85fd3d\"}]},\"type\":\"ConnectorPlacement.EquallySpacedConnector\",\"uuid\":\"206e0d7b-1d35-45e7-9c4c-8a6f9fe9dc79\"}],\"packageUris\":[\"http://schema.mathworks.com/mf0/Connector/R2020b\"],\"version\":\"1.0\"}"
  S6 : Subsystem
      settings: PortSchema="{\"entries\":[{\"content\":{\"sides\":[{\"content\":{\"connectorIds\":[\"In1\"]},\"type\":\"ConnectorPlacement.EquallySpacedRectSide\",\"uuid\":\"4868c43b-8f86-4e2f-a4da-367c2e17d6e4\"},{\"content\":{\"side\":\"RIGHT\"},\"type\":\"ConnectorPlacement.EquallySpacedRectSide\",\"uuid\":\"ebe9b5ec-833b-4a08-98e5-ff684cd7afcb\"},{\"content\":{\"connectorIds\":[\"LConn1\"],\"side\":\"TOP\"},\"type\":\"ConnectorPlacement.EquallySpacedRectSide\",\"uuid\":\"c72df866-8baa-41a8-9bb1-42a4a1fdee71\"},{\"content\":{\"connectorIds\":[\"RConn1\"],\"side\":\"BOTTOM\"},\"type\":\"ConnectorPlacement.EquallySpacedRectSide\",\"uuid\":\"3a9867c5-1563-48cb-a4f4-92deec85fd3d\"}]},\"type\":\"ConnectorPlacement.EquallySpacedConnector\",\"uuid\":\"206e0d7b-1d35-45e7-9c4c-8a6f9fe9dc79\"}],\"packageUris\":[\"http://schema.mathworks.com/mf0/Connector/R2020b\"],\"version\":\"1.0\"}"
  + : PMIOPort  Side=Right
  "~ " : PMIOPort  Port=2  Side=Left
  - : PMIOPort  Port=3  Side=Right
  wires:
  [Sb_c_l] -> Data Type Conversion5/1
  [Sb_b_l] -> Data Type Conversion3/1
  [Sb_a_l] -> Data Type Conversion1/1
  [Sb_a_u] -> Data Type Conversion/1
  [Sb_c_u] -> Data Type Conversion4/1
  [Sb_b_u] -> Data Type Conversion2/1
  Data Type Conversion/1 -> S1/1(g)
  Data Type Conversion1/1 -> S2/1(g)
  Data Type Conversion2/1 -> S3/1(g)
  Data Type Conversion3/1 -> S4/1(g)
  Data Type Conversion4/1 -> S5/1(g)
  Data Type Conversion5/1 -> S6/1(g)
  connections:
  S6/RConn1 -- S4/RConn1 -- S2/RConn1 -- -/RConn1
  S1/LConn1 -- S5/LConn1 -- S3/LConn1 -- +/RConn1
  Phase Splitter/RConn3 -- S6/LConn1 -- S5/RConn1
  Phase Splitter/RConn2 -- S4/LConn1 -- S3/RConn1
  S1/RConn1 -- S2/LConn1 -- Phase Splitter/RConn1
  Phase Splitter/LConn1 -- "~ "/RConn1

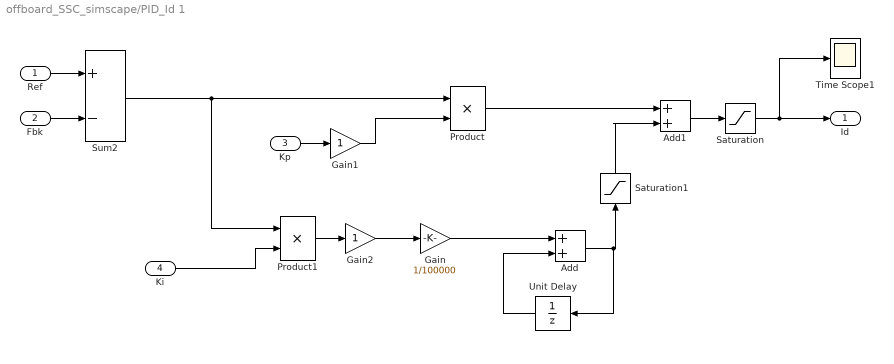
== system offboard_SSC_simscape/PID_Id 1 ==
  Ref : Inport
  Fbk : Inport  Port=2
  Kp : Inport  Port=3
  Ki : Inport  Port=4
  Add : Sum
  Add1 : Sum
  Gain : Gain  Gain=1/100000
  Gain1 : Gain
  Gain2 : Gain
  Product : Product  OutDataTypeStr=Inherit: Same as first input
  Product1 : Product  OutDataTypeStr=Inherit: Same as first input
  Saturation : Saturate  UpperLimit=200  LowerLimit=-200  LinearizeAsGain=off  ZeroCross=off
  Saturation1 : Saturate  UpperLimit=200  LowerLimit=-200  LinearizeAsGain=off  ZeroCross=off
  Sum2 : Sum  Inputs=+-
  Time Scope1 : Scope
      settings: TimeUnits=Metric (based on Time Span)  ActiveDisplayYMinimum=-250  ActiveDisplayYMaximum=250  YLabel=Amplitude  DataLoggingVariableName=ScopeData5
  Unit Delay : UnitDelay  SampleTime=-1  HasFrameUpgradeWarning=on
  Id : Outport
  wires:
  Sum2/1 -> Product1/1, Product/1
  Fbk/1 -> Sum2/2
  Ref/1 -> Sum2/1
  Product1/1 -> Gain2/1
  Add/1 -> Unit Delay/1, Saturation1/1
  Product/1 -> Add1/1
  Gain/1 -> Add/1
  Unit Delay/1 -> Add/2
  Kp/1 -> Gain1/1
  Ki/1 -> Product1/2
  Gain1/1 -> Product/2
  Gain2/1 -> Gain/1
  Add1/1 -> Saturation/1
  Saturation/1 -> Time Scope1/1, Id/1
  Saturation1/1 -> Add1/2

== system offboard_SSC_simscape/PID_Id 2 ==
  Ref : Inport
  Fbk : Inport  Port=2
  Kp : Inport  Port=3
  Ki : Inport  Port=4
  Add : Sum
  Add1 : Sum
  Gain : Gain  Gain=1/100000
  Product : Product  OutDataTypeStr=Inherit: Same as first input
  Product1 : Product  OutDataTypeStr=Inherit: Same as first input
  Saturation : Saturate  UpperLimit=800  LowerLimit=-800  LinearizeAsGain=off  ZeroCross=off
  Saturation1 : Saturate  UpperLimit=800  LowerLimit=-800  ZeroCross=off
  Sum2 : Sum  Inputs=+-
  Time Scope1 : Scope
      settings: TimeUnits=Metric (based on Time Span)  ActiveDisplayYMinimum=-1054.1200630374783  ActiveDisplayYMaximum=796.9605052442555  YLabel=Amplitude  DataLoggingVariableName=ScopeData5
  Unit Delay : UnitDelay  SampleTime=-1  HasFrameUpgradeWarning=on
  Ud : Outport
  wires:
  Add1/1 -> Saturation/1
  Sum2/1 -> Product1/1, Product/1
  Fbk/1 -> Sum2/2
  Ref/1 -> Sum2/1
  Kp/1 -> Product/2
  Ki/1 -> Product1/2
  Product1/1 -> Gain/1
  Add/1 -> Unit Delay/1, Saturation1/1
  Product/1 -> Add1/1
  Saturation/1 -> Time Scope1/1, Ud/1
  Gain/1 -> Add/1
  Unit Delay/1 -> Add/2
  Saturation1/1 -> Add1/2

== system offboard_SSC_simscape/PID_Iq 3 ==
  Ref : Inport
  Fbk : Inport  Port=2
  Kp : Inport  Port=3
  Ki : Inport  Port=4
  Add : Sum
  Add1 : Sum
  Gain : Gain  Gain=1/100000
  Product : Product  OutDataTypeStr=Inherit: Same as first input
  Product1 : Product  OutDataTypeStr=Inherit: Same as first input
  Saturation : Saturate  UpperLimit=800  LowerLimit=-800  LinearizeAsGain=off  ZeroCross=off
  Saturation1 : Saturate  UpperLimit=800  LowerLimit=-800  LinearizeAsGain=off  ZeroCross=off
  Sum2 : Sum  Inputs=+-
  Time Scope1 : Scope
      settings: TimeUnits=Metric (based on Time Span)  ActiveDisplayYMinimum=-295.24637  ActiveDisplayYMaximum=1032.80515  YLabel=Amplitude  DataLoggingVariableName=ScopeData6
  Unit Delay : UnitDelay  SampleTime=-1  HasFrameUpgradeWarning=on
  Uq : Outport
  wires:
  Add1/1 -> Saturation/1
  Sum2/1 -> Product1/1, Product/1
  Fbk/1 -> Sum2/2
  Ref/1 -> Sum2/1
  Kp/1 -> Product/2
  Ki/1 -> Product1/2
  Product1/1 -> Gain/1
  Add/1 -> Unit Delay/1, Saturation1/1
  Product/1 -> Add1/1
  Gain/1 -> Add/1
  Unit Delay/1 -> Add/2
  Saturation/1 -> Time Scope1/1, Uq/1
  Saturation1/1 -> Add1/2

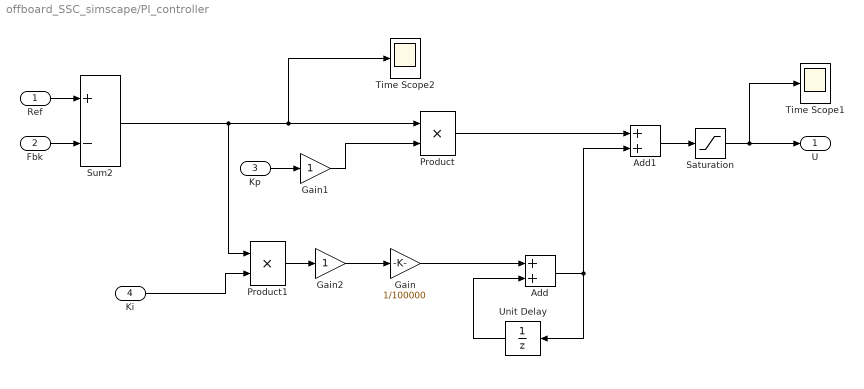
== system offboard_SSC_simscape/PI_controller ==
  Ref : Inport
  Fbk : Inport  Port=2
  Kp : Inport  Port=3
  Ki : Inport  Port=4
  Add : Sum
  Add1 : Sum
  Gain : Gain  Gain=1/100000
  Gain1 : Gain
  Gain2 : Gain
  Product : Product  OutDataTypeStr=Inherit: Same as first input
  Product1 : Product  OutDataTypeStr=Inherit: Same as first input
  Saturation : Saturate  UpperLimit=400  LowerLimit=-400  LinearizeAsGain=off  ZeroCross=off
  Sum2 : Sum  Inputs=+-
  Time Scope1 : Scope
      settings: TimeUnits=Metric (based on Time Span)  ActiveDisplayYMinimum=-500  ActiveDisplayYMaximum=500  YLabel=Amplitude  DataLoggingVariableName=ScopeData5
  Time Scope2 : Scope
      settings: TimeUnits=Metric (based on Time Span)  ActiveDisplayYMinimum=-48.22028  ActiveDisplayYMaximum=227.58003  YLabel=Amplitude  DataLoggingVariableName=ScopeData6
  Unit Delay : UnitDelay  SampleTime=-1  HasFrameUpgradeWarning=on
  U : Outport
  wires:
  Fbk/1 -> Sum2/2
  Ref/1 -> Sum2/1
  Product1/1 -> Gain2/1
  Add/1 -> Unit Delay/1, Add1/2
  Product/1 -> Add1/1
  Gain/1 -> Add/1
  Unit Delay/1 -> Add/2
  Ki/1 -> Product1/2
  Gain2/1 -> Gain/1
  Add1/1 -> Saturation/1
  Saturation/1 -> Time Scope1/1, U/1
  Kp/1 -> Gain1/1
  Gain1/1 -> Product/2
  Sum2/1 -> Product1/1, Time Scope2/1, Product/1

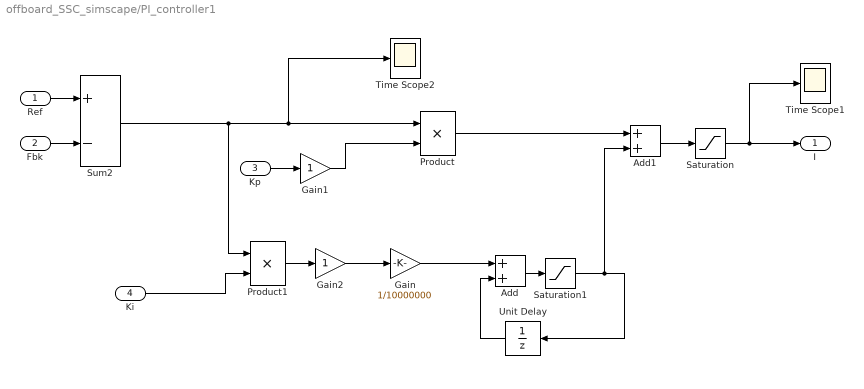
== system offboard_SSC_simscape/PI_controller1 ==
  Ref : Inport
  Fbk : Inport  Port=2
  Kp : Inport  Port=3
  Ki : Inport  Port=4
  Add : Sum
  Add1 : Sum
  Gain : Gain  Gain=1/10000000
  Gain1 : Gain
  Gain2 : Gain
  Product : Product  OutDataTypeStr=Inherit: Same as first input
  Product1 : Product  OutDataTypeStr=Inherit: Same as first input
  Saturation : Saturate  UpperLimit=50  LowerLimit=0  LinearizeAsGain=off  ZeroCross=off
  Saturation1 : Saturate  UpperLimit=50  LowerLimit=-50  LinearizeAsGain=off  ZeroCross=off
  Sum2 : Sum  Inputs=+-
  Time Scope1 : Scope
      settings: TimeUnits=Metric (based on Time Span)  ActiveDisplayYMinimum=10.50458  ActiveDisplayYMaximum=21.05505  YLabel=Amplitude  DataLoggingVariableName=ScopeData5
  Time Scope2 : Scope
      settings: TimeUnits=Metric (based on Time Span)  ActiveDisplayYMinimum=-48.22028  ActiveDisplayYMaximum=227.58003  YLabel=Amplitude  DataLoggingVariableName=ScopeData6
  Unit Delay : UnitDelay  InitialCondition=0.9  SampleTime=-1  HasFrameUpgradeWarning=on
  I : Outport
  wires:
  Fbk/1 -> Sum2/2
  Ref/1 -> Sum2/1
  Product1/1 -> Gain2/1
  Product/1 -> Add1/1
  Gain/1 -> Add/1
  Unit Delay/1 -> Add/2
  Ki/1 -> Product1/2
  Gain2/1 -> Gain/1
  Add1/1 -> Saturation/1
  Saturation/1 -> Time Scope1/1, I/1
  Kp/1 -> Gain1/1
  Gain1/1 -> Product/2
  Sum2/1 -> Product1/1, Time Scope2/1, Product/1
  Add/1 -> Saturation1/1
  Saturation1/1 -> Add1/2, Unit Delay/1

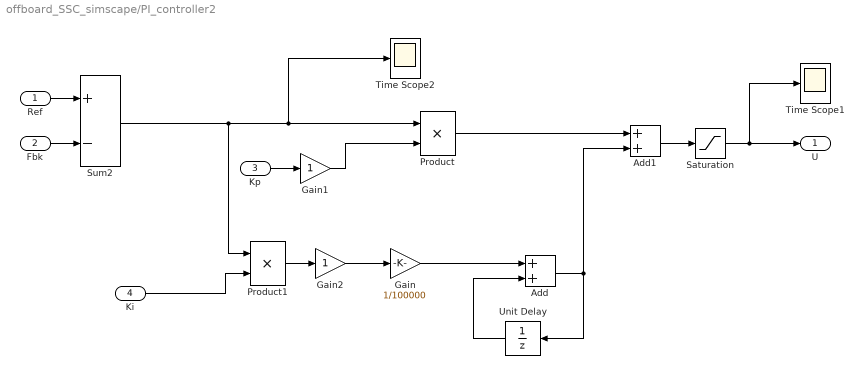
== system offboard_SSC_simscape/PI_controller2 ==
  Ref : Inport
  Fbk : Inport  Port=2
  Kp : Inport  Port=3
  Ki : Inport  Port=4
  Add : Sum
  Add1 : Sum
  Gain : Gain  Gain=1/100000
  Gain1 : Gain
  Gain2 : Gain
  Product : Product  OutDataTypeStr=Inherit: Same as first input
  Product1 : Product  OutDataTypeStr=Inherit: Same as first input
  Saturation : Saturate  UpperLimit=400  LowerLimit=-400  LinearizeAsGain=off  ZeroCross=off
  Sum2 : Sum  Inputs=+-
  Time Scope1 : Scope
      settings: TimeUnits=Metric (based on Time Span)  ActiveDisplayYMinimum=-500  ActiveDisplayYMaximum=500  YLabel=Amplitude  DataLoggingVariableName=ScopeData5
  Time Scope2 : Scope
      settings: TimeUnits=Metric (based on Time Span)  ActiveDisplayYMinimum=-48.22028  ActiveDisplayYMaximum=227.58003  YLabel=Amplitude  DataLoggingVariableName=ScopeData6
  Unit Delay : UnitDelay  SampleTime=-1  HasFrameUpgradeWarning=on
  U : Outport
  wires:
  Fbk/1 -> Sum2/2
  Ref/1 -> Sum2/1
  Product1/1 -> Gain2/1
  Add/1 -> Unit Delay/1, Add1/2
  Product/1 -> Add1/1
  Gain/1 -> Add/1
  Unit Delay/1 -> Add/2
  Ki/1 -> Product1/2
  Gain2/1 -> Gain/1
  Add1/1 -> Saturation/1
  Saturation/1 -> Time Scope1/1, U/1
  Kp/1 -> Gain1/1
  Gain1/1 -> Product/2
  Sum2/1 -> Product1/1, Time Scope2/1, Product/1

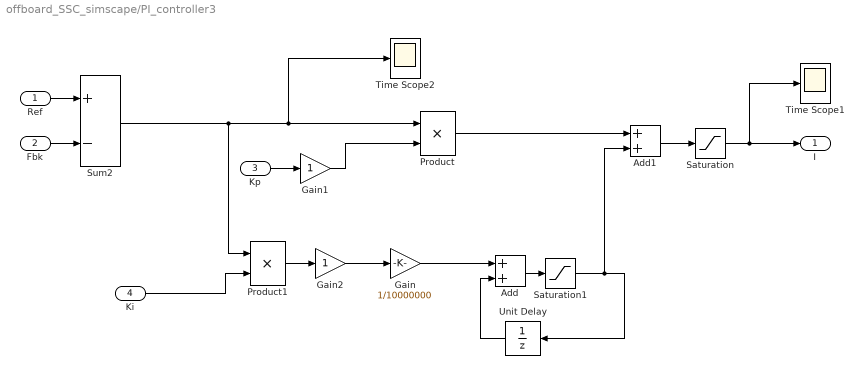
== system offboard_SSC_simscape/PI_controller3 ==
  Ref : Inport
  Fbk : Inport  Port=2
  Kp : Inport  Port=3
  Ki : Inport  Port=4
  Add : Sum
  Add1 : Sum
  Gain : Gain  Gain=1/10000000
  Gain1 : Gain
  Gain2 : Gain
  Product : Product  OutDataTypeStr=Inherit: Same as first input
  Product1 : Product  OutDataTypeStr=Inherit: Same as first input
  Saturation : Saturate  UpperLimit=50  LowerLimit=0  LinearizeAsGain=off  ZeroCross=off
  Saturation1 : Saturate  UpperLimit=50  LowerLimit=-50  LinearizeAsGain=off  ZeroCross=off
  Sum2 : Sum  Inputs=+-
  Time Scope1 : Scope
      settings: TimeUnits=Metric (based on Time Span)  ActiveDisplayYMinimum=10.50458  ActiveDisplayYMaximum=21.05505  YLabel=Amplitude  DataLoggingVariableName=ScopeData5
  Time Scope2 : Scope
      settings: TimeUnits=Metric (based on Time Span)  ActiveDisplayYMinimum=-48.22028  ActiveDisplayYMaximum=227.58003  YLabel=Amplitude  DataLoggingVariableName=ScopeData6
  Unit Delay : UnitDelay  InitialCondition=0.9  SampleTime=-1  HasFrameUpgradeWarning=on
  I : Outport
  wires:
  Fbk/1 -> Sum2/2
  Ref/1 -> Sum2/1
  Product1/1 -> Gain2/1
  Product/1 -> Add1/1
  Gain/1 -> Add/1
  Unit Delay/1 -> Add/2
  Ki/1 -> Product1/2
  Gain2/1 -> Gain/1
  Add1/1 -> Saturation/1
  Saturation/1 -> Time Scope1/1, I/1
  Kp/1 -> Gain1/1
  Gain1/1 -> Product/2
  Sum2/1 -> Product1/1, Time Scope2/1, Product/1
  Add/1 -> Saturation1/1
  Saturation1/1 -> Add1/2, Unit Delay/1

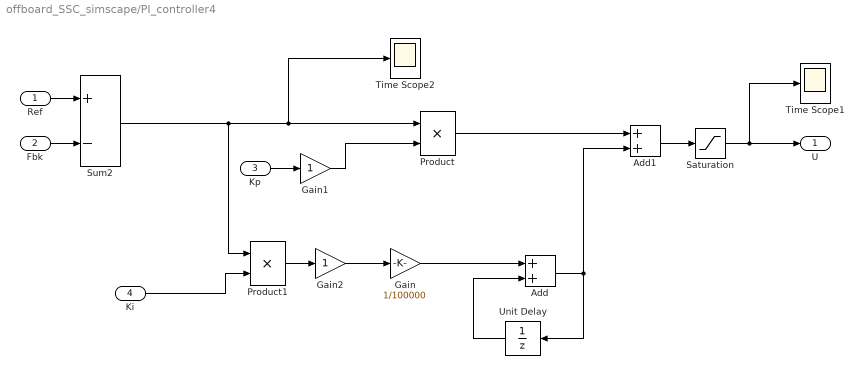
== system offboard_SSC_simscape/PI_controller4 ==
  Ref : Inport
  Fbk : Inport  Port=2
  Kp : Inport  Port=3
  Ki : Inport  Port=4
  Add : Sum
  Add1 : Sum
  Gain : Gain  Gain=1/100000
  Gain1 : Gain
  Gain2 : Gain
  Product : Product  OutDataTypeStr=Inherit: Same as first input
  Product1 : Product  OutDataTypeStr=Inherit: Same as first input
  Saturation : Saturate  UpperLimit=400  LowerLimit=-400  LinearizeAsGain=off  ZeroCross=off
  Sum2 : Sum  Inputs=+-
  Time Scope1 : Scope
      settings: TimeUnits=Metric (based on Time Span)  ActiveDisplayYMinimum=-500  ActiveDisplayYMaximum=500  YLabel=Amplitude  DataLoggingVariableName=ScopeData5
  Time Scope2 : Scope
      settings: TimeUnits=Metric (based on Time Span)  ActiveDisplayYMinimum=-48.22028  ActiveDisplayYMaximum=227.58003  YLabel=Amplitude  DataLoggingVariableName=ScopeData6
  Unit Delay : UnitDelay  SampleTime=-1  HasFrameUpgradeWarning=on
  U : Outport
  wires:
  Fbk/1 -> Sum2/2
  Ref/1 -> Sum2/1
  Product1/1 -> Gain2/1
  Add/1 -> Unit Delay/1, Add1/2
  Product/1 -> Add1/1
  Gain/1 -> Add/1
  Unit Delay/1 -> Add/2
  Ki/1 -> Product1/2
  Gain2/1 -> Gain/1
  Add1/1 -> Saturation/1
  Saturation/1 -> Time Scope1/1, U/1
  Kp/1 -> Gain1/1
  Gain1/1 -> Product/2
  Sum2/1 -> Product1/1, Time Scope2/1, Product/1

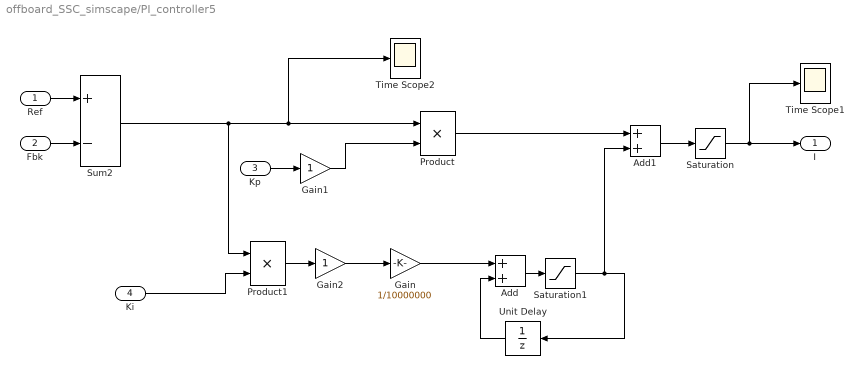
== system offboard_SSC_simscape/PI_controller5 ==
  Ref : Inport
  Fbk : Inport  Port=2
  Kp : Inport  Port=3
  Ki : Inport  Port=4
  Add : Sum
  Add1 : Sum
  Gain : Gain  Gain=1/10000000
  Gain1 : Gain
  Gain2 : Gain
  Product : Product  OutDataTypeStr=Inherit: Same as first input
  Product1 : Product  OutDataTypeStr=Inherit: Same as first input
  Saturation : Saturate  UpperLimit=50  LowerLimit=0  LinearizeAsGain=off  ZeroCross=off
  Saturation1 : Saturate  UpperLimit=50  LowerLimit=-50  LinearizeAsGain=off  ZeroCross=off
  Sum2 : Sum  Inputs=+-
  Time Scope1 : Scope
      settings: TimeUnits=Metric (based on Time Span)  ActiveDisplayYMinimum=10.50458  ActiveDisplayYMaximum=21.05505  YLabel=Amplitude  DataLoggingVariableName=ScopeData5
  Time Scope2 : Scope
      settings: TimeUnits=Metric (based on Time Span)  ActiveDisplayYMinimum=-48.22028  ActiveDisplayYMaximum=227.58003  YLabel=Amplitude  DataLoggingVariableName=ScopeData6
  Unit Delay : UnitDelay  InitialCondition=0.9  SampleTime=-1  HasFrameUpgradeWarning=on
  I : Outport
  wires:
  Fbk/1 -> Sum2/2
  Ref/1 -> Sum2/1
  Product1/1 -> Gain2/1
  Product/1 -> Add1/1
  Gain/1 -> Add/1
  Unit Delay/1 -> Add/2
  Ki/1 -> Product1/2
  Gain2/1 -> Gain/1
  Add1/1 -> Saturation/1
  Saturation/1 -> Time Scope1/1, I/1
  Kp/1 -> Gain1/1
  Gain1/1 -> Product/2
  Sum2/1 -> Product1/1, Time Scope2/1, Product/1
  Add/1 -> Saturation1/1
  Saturation1/1 -> Add1/2, Unit Delay/1

== system offboard_SSC_simscape/PLL (3ph) ==
  abc : Inport
  "Sinusoidal Measurement (PLL, Three-Phase)" : eeSinusoidalMeasurement/Sinusoidal Measurement (PLL, Three-Phase)  Kp_LF=5  Ki_LF=1000  F0=60  Theta0=PLL_3ph__class([0 60]).objParamMappingDerived.NewDerivedParam.Theta0  Ts=0.0001
  Terminator : Terminator
  Freq : Outport  VectorParamsAs1DForOutWhenUnconnected=off
  wt : Outport  Port=2  VectorParamsAs1DForOutWhenUnconnected=off
  wires:
  "Sinusoidal Measurement (PLL, Three-Phase)"/3 -> Terminator/1
  "Sinusoidal Measurement (PLL, Three-Phase)"/2 -> wt/1
  "Sinusoidal Measurement (PLL, Three-Phase)"/1 -> Freq/1
  abc/1 -> "Sinusoidal Measurement (PLL, Three-Phase)"/1

== system offboard_SSC_simscape/Subsystem ==
  PS-Simulink Converter2 : nesl_utility/PS-Simulink Converter  PhysicalDomain=network_engine_domain  SubClassName=ps_output  LeftPortType=input  RightPortType=output  PseudoPeriodic=off  Frequencies=[]  VectorFormat=inherit  Unit=inherit  AffineConversion=off
  Unit Delay1 : UnitDelay  SampleTime=-1  HasFrameUpgradeWarning=on
  Voltage Sensor : fl_lib/Electrical/Electrical Sensors/Voltage Sensor
  + : PMIOPort  Side=Left
  - : PMIOPort  Port=2  Side=Right
  V : Outport
  wires:
  PS-Simulink Converter2/1 -> Unit Delay1/1
  Unit Delay1/1 -> V/1
  connections:
  Voltage Sensor/LConn1 -- +/RConn1
  PS-Simulink Converter2/LConn1 -- Voltage Sensor/RConn1
  Voltage Sensor/RConn2 -- -/RConn1
